simulink model "SimulinkModel"  (R2022b)
settings: Solver=VariableStepAuto  StartTime=0.0  StopTime=500  RelTol=1e-3
model workspace (MAT data in the model file):
  E = 1
  Mc = 2
  Mt = 1
  g = 9.81
  k = 1
  lamda = 0.03
settings Model: Creator=abuba  LastModifiedBy=abuba

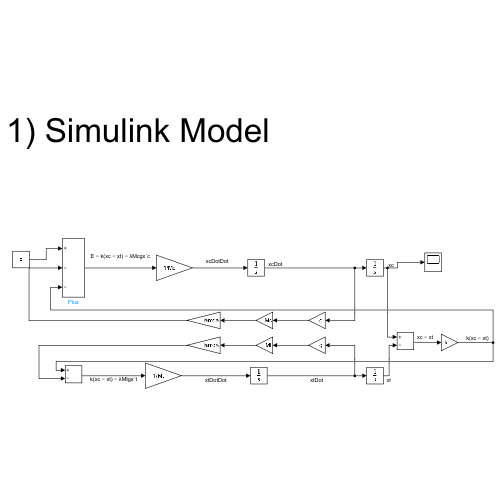
[thumbnail: Simulink's stored preview of the top-level diagram]
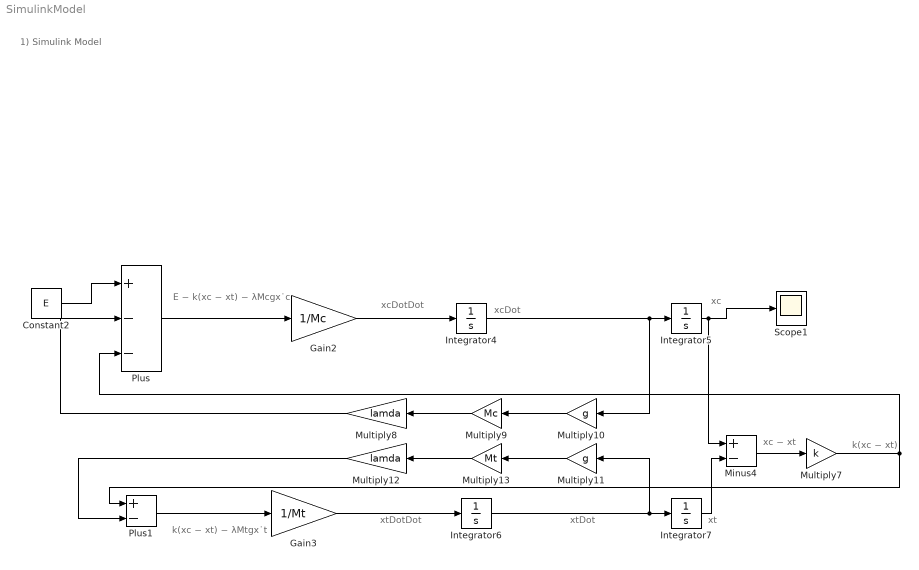
== system SimulinkModel ==
  note: 1) Simulink Model
  note: k(xc − xt) − λMtgx˙t
  note: E − k(xc − xt) − λMcgx˙c
  note: k(xc − xt)
  note: xc − xt
  note: xcDotDot
  note: xcDot
  note: xc
  note: xt
  note: xtDot
  note: xtDotDot
  Constant2 : Constant  Value=E
  Gain2 : Gain  Gain=1/Mc
  Gain3 : Gain  Gain=1/Mt
  Integrator{4..7} (4 alike) : Integrator
  Minus4 : Sum  Inputs=+-
  Multiply10 : Gain  Gain=g
  Multiply11 : Gain  Gain=g
  Multiply12 : Gain  Gain=lamda
  Multiply13 : Gain  Gain=Mt
  Multiply7 : Gain  Gain=k
  Multiply8 : Gain  Gain=lamda
  Multiply9 : Gain  Gain=Mc
  Plus : Sum  Inputs=+--
  Plus1 : Sum  Inputs=+-
  Scope1 : Scope
  wires:
  Integrator4/1 -> Integrator5/1, Multiply10/1
  Integrator5/1 -> Scope1/1, Minus4/1
  Integrator6/1 -> Integrator7/1, Multiply11/1
  Gain3/1 -> Integrator6/1
  Integrator7/1 -> Minus4/2
  Minus4/1 -> Multiply7/1
  Multiply10/1 -> Multiply9/1
  Multiply9/1 -> Multiply8/1
  Multiply13/1 -> Multiply12/1
  Multiply11/1 -> Multiply13/1
  Plus/1 -> Gain2/1
  Multiply8/1 -> Plus/2
  Constant2/1 -> Plus/1
  Plus1/1 -> Gain3/1
  Multiply12/1 -> Plus1/2
  Gain2/1 -> Integrator4/1
  Multiply7/1 -> Plus/3, Plus1/1
